simulink model "lab12"  (R2017a)
settings: Solver=VariableStepAuto  StartTime=0.0  StopTime=10.0  RelTol=1e-3
InitFcn:
  | f
settings Model: Creator=Peter  LastModifiedBy=Peter

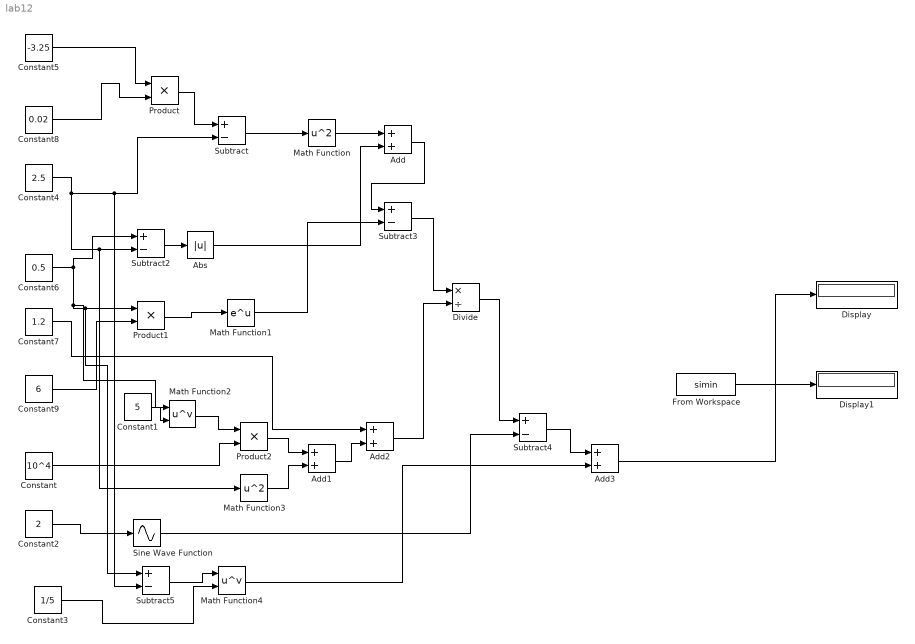
== system lab12 ==
  Abs : Abs
  Add{,1..3} (4 alike) : Sum
  Constant : Constant  Value=10^4
  Constant1 : Constant  Value=5
  Constant2 : Constant  Value=2
  Constant3 : Constant  Value=1/5
  Constant4 : Constant  Value=2.5
  Constant5 : Constant  Value=-3.25
  Constant6 : Constant  Value=0.5
  Constant7 : Constant  Value=1.2
  Constant8 : Constant  Value=0.02
  Constant9 : Constant  Value=6
  Display : Display
  Display1 : Display
  Divide : Product  Inputs=*/
  From Workspace : FromWorkspace  VariableName=simin  Interpolate=off  OutputAfterFinalValue=Holding final value
  Math Function : Math  Operator=square  SaturateOnIntegerOverflow=on
  Math Function1 : Math  SaturateOnIntegerOverflow=on
  Math Function2 : Math  Operator=pow  SaturateOnIntegerOverflow=on
  Math Function3 : Math  Operator=square  SaturateOnIntegerOverflow=on
  Math Function4 : Math  Operator=pow  SaturateOnIntegerOverflow=on
  Product : Product
  Product1 : Product
  Product2 : Product
  Sine Wave Function : Sin  TimeSource=Use external signal  SampleTime=0
  Subtract{,2..5} (5 alike) : Sum  Inputs=+-
  wires:
  From Workspace/1 -> Display1/1
  Constant8/1 -> Product/2
  Constant5/1 -> Product/1
  Product/1 -> Subtract/1
  Subtract/1 -> Math Function/1
  Math Function/1 -> Add/1
  Subtract2/1 -> Abs/1
  Abs/1 -> Add/2
  Constant9/1 -> Product1/2
  Product1/1 -> Math Function1/1
  Add/1 -> Subtract3/1
  Math Function1/1 -> Subtract3/2
  Constant1/1 -> Math Function2/2
  Math Function2/1 -> Product2/1
  Constant/1 -> Product2/2
  Math Function3/1 -> Add1/2
  Product2/1 -> Add1/1
  Add1/1 -> Add2/2
  Constant7/1 -> Add2/1
  Add2/1 -> Divide/2
  Subtract3/1 -> Divide/1
  Divide/1 -> Subtract4/1
  Constant4/1 -> Math Function3/1, Subtract2/2, Subtract5/2, Subtract/2
  Subtract5/1 -> Math Function4/1
  Subtract4/1 -> Add3/1
  Math Function4/1 -> Add3/2
  Add3/1 -> Display/1
  Constant6/1 -> Subtract2/1, Math Function2/1, Subtract5/1, Product1/1
  Constant3/1 -> Math Function4/2
  Sine Wave Function/1 -> Subtract4/2
  Constant2/1 -> Sine Wave Function/1
